simulink model "model"  (R2018a)
settings: Solver=VariableStepAuto  StartTime=0.0  StopTime=model_time  MaxStep=0.01  RelTol=1e-3
undefined symbols (not defined in the file): a0, b0, b1, const_sourse
libraries: simulink_extras x2
settings Model: Creator=Asus  LastModifiedBy=Asus

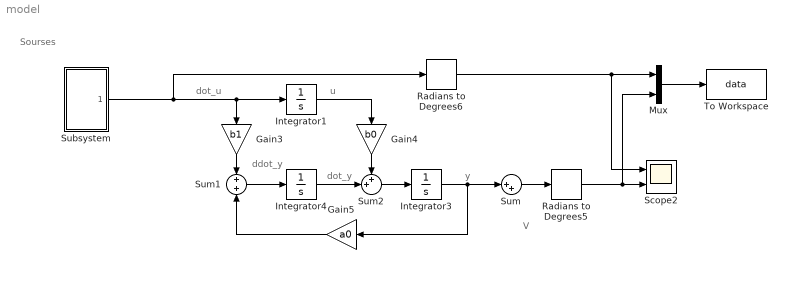
== system model ==
  note: V
  note: y
  note: ddot_y
  note: dot_u
  note: Sourses
  note: u
  note: dot_y
  Gain3 : Gain  Gain=b1
  Gain4 : Gain  Gain=b0
  Gain5 : Gain  Gain=a0
  Integrator1 : Integrator
  Integrator3 : Integrator
  Integrator4 : Integrator
  Mux : Mux  Inputs=2
  Radians to Degrees5 : simulink_extras/Transformations/Radians to Degrees
  Radians to Degrees6 : simulink_extras/Transformations/Radians to Degrees
  Scope2 : Scope  NumInputPorts=2
  Subsystem : Subsystem
  Sum : Sum  Inputs=|++
  Sum1 : Sum
  Sum2 : Sum  Inputs=++|
  To Workspace : ToWorkspace  VariableName=data  SampleTime=-1
  wires:
  Sum1/1 -> Integrator4/1
  Integrator4/1 -> Sum2/2
  Sum2/1 -> Integrator3/1
  Integrator3/1 -> Gain5/1, Sum/1
  Radians to Degrees6/1 -> Mux/1, Scope2/1
  Gain5/1 -> Sum1/2
  Mux/1 -> To Workspace/1
  Radians to Degrees5/1 -> Mux/2, Scope2/2
  Subsystem/1(sources) -> Integrator1/1, Gain3/1, Radians to Degrees6/1
  Sum/1 -> Radians to Degrees5/1
  Gain3/1 -> Sum1/1
  Gain4/1 -> Sum2/1
  Integrator1/1 -> Gain4/1
  ? -> Sum/2

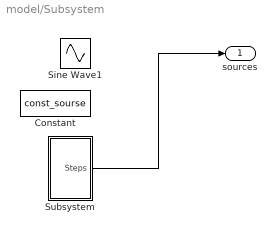
== system model/Subsystem ==
  Constant : Constant  Value=const_sourse
  Sine Wave1 : Sin  Amplitude=0.3  Frequency=0.1  SampleTime=0
  Subsystem : Subsystem
  sources : Outport
  wires:
  Subsystem/1(Steps) -> sources/1

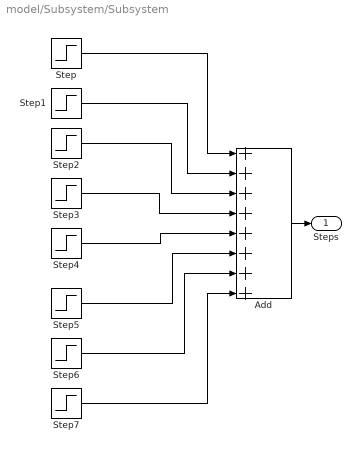
== system model/Subsystem/Subsystem ==
  Add : Sum  Inputs=++++++++
  Step : Step  After=0.1  SampleTime=0
  Step1 : Step  Time=2  After=-0.2  SampleTime=0
  Step2 : Step  Time=4  After=0.15  SampleTime=0
  Step3 : Step  Time=5  After=-0.05  SampleTime=0
  Step4 : Step  Time=7  After=0.1  SampleTime=0
  Step5 : Step  Time=9  After=-0.15  SampleTime=0
  Step6 : Step  Time=10  After=0.025  SampleTime=0
  Step7 : Step  Time=11  After=0.025  SampleTime=0
  Steps : Outport
  wires:
  Step7/1 -> Add/8
  Step1/1 -> Add/2
  Add/1 -> Steps/1
  Step/1 -> Add/1
  Step2/1 -> Add/3
  Step4/1 -> Add/5
  Step3/1 -> Add/4
  Step6/1 -> Add/7
  Step5/1 -> Add/6
